simulink model "Echo"  (R2020a)
settings: Solver=VariableStepAuto  StartTime=0.0  StopTime=inf  RelTol=1e-3
libraries: audiosources x1, dspsnks4 x1, simulink x1
settings Model: Creator=Zach Jones  LastModifiedBy=Zach Jones

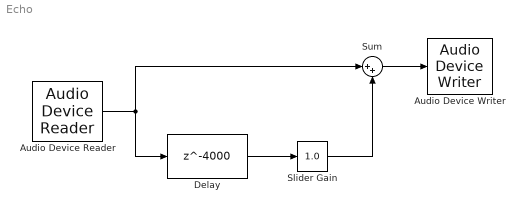
== system Echo ==
  Audio Device Reader : audiosources/Audio Device Reader  Driver=DirectSound  Device=Microphone (iMic USB audio system)  SampleRate=44100  NumChannels=1  SamplesPerFrame=1024  BitDepth=16-bit integer  NumBuffers=10  DefaultInputChannelMapping=on  InputChannelMapping=1:2  OutputNumOverrunSamples=off  OutputDataType=double  DriverIdx=1  DeviceWarnFlag=''
      settings: SourceProductBaseCode=AU
  Audio Device Writer : dspsnks4/Audio Device Writer  Driver=DirectSound  Device=Headphones (Realtek(R) Audio)  InheritSampleRate=on  SampleRate=44100  BitDepth=16-bit integer  BufferSize=4096  NumBuffers=10  DefaultOutputChannelMapping=on  OutputChannelMapping=1:2  OutputNumUnderrunSamples=off  DriverIdx=1  DeviceWarnFlag=''
  Delay : Delay  DelayLength=4000  InputProcessing=Columns as channels (frame based)
  Slider Gain : simulink/Math Operations/Slider Gain  gain=1.0  low=0  high=1
  Sum : Sum  Inputs=|++
  wires:
  Sum/1 -> Audio Device Writer/1
  Audio Device Reader/1 -> Sum/1, Delay/1
  Delay/1 -> Slider Gain/1
  Slider Gain/1 -> Sum/2
